simulink library "EVComponents_utility_lib"  (R2021a)
settings: Solver=VariableStepAuto  StartTime=0.0  StopTime=10.0  RelTol=1e-3
undefined symbols (not defined in the file): DiscIntNeverNeededParam
libraries: fl_lib x7, nesl_utility x5, $bdroot x1, sdl_lib x1
settings Model: Creator=isaacito  LastModifiedBy=isaacito
settings SolverCC: AlgebraicLoopSolver=TrustRegion
settings DebuggingCC: SFMachineParentedDataDiag=warning

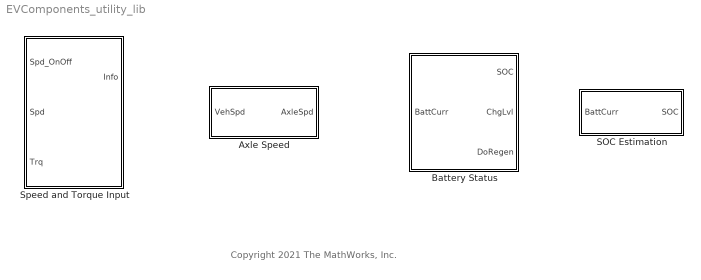
== system EVComponents_utility_lib ==
  note: Copyright 2021 The MathWorks, Inc.
  Axle Speed : Subsystem  mask(Vehicle Speed to Axle Speed){Value=0.3}
      mask prompts: Value "Tire Rolling Radius [m]"
      mask help: Given longitudinal vehicle speed, this block computes the axle rotational speed.
      mask TypeOptions Value: Tire Rolling Radius (m)/Value
  Battery Status : Subsystem  mask(Battery Status){capacity_kWh=40, voltagePerCell_V=3.5, initial_SOC_pct=98, SocHigh=95, SocLow=50, SocEmpty=6}
      mask prompts: capacity_kWh "Battery Capacity [kW*hr]"; voltagePerCell_V "Voltage per cell [V]"; initial_SOC_pct "Initial SOC [%]"; SocHigh "SOC High-Mid Threshold [%]"; SocLow "SOC Mid-Low Threshold [%]"; SocEmpty "SOC Low-Empty Threshold [%]"
      mask help:
      | Battery current input assumes that the negative (positive) value current means consuming (charging) electric power from (to) the battery.
      |
      | SOC outport outputs the state of charge of the battery in %.
      |
      | ChgLvl outport outputs the charge levels 0 (empty), 1 (low), 2 (mid), or 3 (high). Specify thresholds in SOC Threshold parameters.
      |
      | DoRegen outport outputs true for empty/low/mid battery charge level and false for high. Use this signal to avoid overcharging the battery.
      mask init:
      | if initial_SOC_pct > SocHigh
      |   initialChgLvl = 3;
      | elseif initial_SOC_pct < SocEmpty
      |   initialChgLvl = 0;
      | elseif initial_SOC_pct > SocLow
      |   initialChgLvl = 2;
      | else
      |   initialChgLvl = 1;
      | end
      mask TypeOptions capacity_kWh: SOC Estimation/capacity_kWh
      mask TypeOptions voltagePerCell_V: SOC Estimation/voltagePerCell_V
      mask TypeOptions initial_SOC_pct: SOC Estimation/initial_SOC_pct
      mask DialogControl Container2 Prompt: Parameters
  SOC Estimation : Subsystem  mask(Battery State-of-Charge Estimation){capacity_kWh=10, voltagePerCell_V=3.5, initial_SOC_pct=90}
      mask prompts: capacity_kWh "Battery Capacity [kW*hr]"; voltagePerCell_V "Voltage per cell [V]"; initial_SOC_pct "Initial SOC [%]"
      mask help: Battery current input assumes that the negative value current meas consuming electric power from the battery.
      mask TypeOptions capacity_kWh: Capacity (kW*hr)/Value
      mask TypeOptions voltagePerCell_V: Voltage per Cell (V)/Value
      mask TypeOptions initial_SOC_pct: Initial SOC (%)/Value
  Speed and Torque Input : Subsystem  mask(Speed and Torque Input){t_friction=10000, t_locked=10000, w_tol=0.001, initial_state_locked=sdl.enum.initial_lock.unlocked}
      mask prompts: t_friction "Kinetic friction torque [N*m]"; t_locked "Static friction torque [N*m]"; w_tol "Clutch velocity tolerance [rad/s]"; initial_state_locked "Initial state"
      mask help:
      | This block acts as angular speed and torque source for Simscape Mechanical Rotational connection. Pass 0 or 1 at Spd_OnOff inport to disable or enable speed input Spd, respectively.
      |
      | Spd inport takes angular speed in rpm. Trq inport takes torques in N*m. Node R is Simscape Mechanical Rotational connection node. Info outport outputs angular speed and torque at R.
      |
      | Block parameters correspond to the Logic-Controlled Clutch block in Simscape Driveline.
      mask TypeOptions t_friction:
      | Logic-Controlled
      | Clutch/t_friction
      mask TypeOptions t_locked:
      | Logic-Controlled
      | Clutch/t_locked
      mask TypeOptions w_tol:
      | Logic-Controlled
      | Clutch/w_tol
      mask TypeOptions initial_state_locked:
      | Logic-Controlled
      | Clutch/initial_state_locked

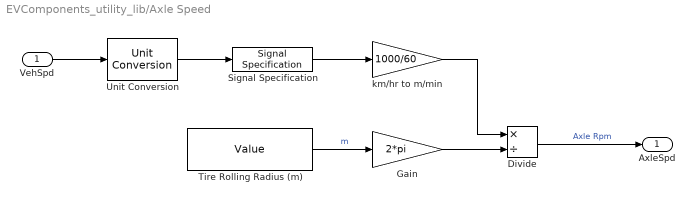
== system EVComponents_utility_lib/Axle Speed ==
  VehSpd : Inport
      settings: AttributesFormatString=%<Unit>
  Divide : Product  Inputs=*/
  Gain : Gain  Gain=2*pi
  Signal Specification : SignalSpecification  Unit=km/hr
  Tire Rolling Radius (m) : Constant  Value=Value
  Unit Conversion : UnitConversion
  km/hr to m/min : Gain  Gain=1000/60
  AxleSpd : Outport  Unit=rpm  VectorParamsAs1DForOutWhenUnconnected=off
      settings: AttributesFormatString=%<Unit>
  wires:
  Tire Rolling Radius (m)/1 -> Gain/1  "m"
  Gain/1 -> Divide/2
  Divide/1 -> AxleSpd/1  "Axle Rpm"
  Unit Conversion/1 -> Signal Specification/1
  VehSpd/1 -> Unit Conversion/1
  Signal Specification/1 -> km/hr to m/min/1
  km/hr to m/min/1 -> Divide/1

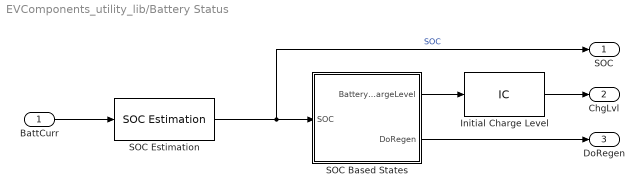
== system EVComponents_utility_lib/Battery Status ==
  BattCurr : Inport
  Initial Charge Level : InitialCondition  Value=initialChgLvl
  SOC Based States : Stateflow chart  TreatAsAtomicUnit=on
      settings: PortSchema="{\"entries\":[{\"content\":{\"sides\":[{\"content\":{\"connectorIds\":[\"In1\"]},\"type\":\"ConnectorPlacement.EquallySpacedRectSide\",\"uuid\":\"6842a8e0-1533-443f-9239-a32cee073609\"},{\"content\":{\"connectorIds\":[\"Out2\",\"Out1\"],\"side\":\"RIGHT\"},\"type\":\"ConnectorPlacement.EquallySpacedRectSide\",\"uuid\":\"4d5668fa-96aa-414a-86e2-97093b53d80f\"},{\"content\":{\"connectorIds\":[],\"side\":\"TOP\"},\"type\":\"ConnectorPlacement.EquallySpacedRectSide\",\"uuid\":\"b14b12e5-8ddb-4090-8868-1deded7232d1\"},{\"content\":{\"connectorIds\":[],\"side\":\"HIDDEN\"},\"type\":\"ConnectorPlacement.EquallySpacedRectSide\",\"uuid\":\"15641086-7bcd-4523-b266-ad823dacae84\"}]},\"type\":\"ConnectorPlacement.EquallySpacedConnector\",\"uuid\":\"9c75feda-b5f3-44ec-8ad2-652491ceb2eb\"}],\"packageUris\":[\"http://schema.mathworks.com/mf0/Connector/R2020b\"],\"version\":\"1.0\"}"
  SOC Estimation : $bdroot/SOC Estimation  capacity_kWh=capacity_kWh  voltagePerCell_V=voltagePerCell_V  initial_SOC_pct=initial_SOC_pct
  SOC : Outport
  ChgLvl : Outport  Port=2
  DoRegen : Outport  Port=3
  wires:
  SOC Estimation/1 -> SOC/1, SOC Based States/1(SOC)  "SOC"
  SOC Based States/1(DoRegen) -> DoRegen/1
  SOC Based States/2(BatteryChargeLevel) -> Initial Charge Level/1
  BattCurr/1 -> SOC Estimation/1
  Initial Charge Level/1 -> ChgLvl/1

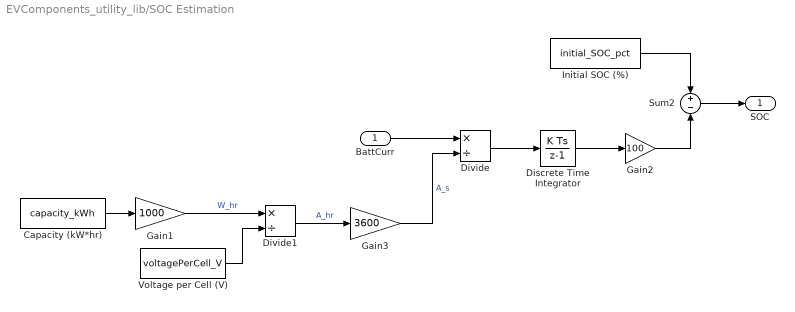
== system EVComponents_utility_lib/SOC Estimation ==
  BattCurr : Inport  Unit=A
      settings: AttributesFormatString=%<Unit>
  Capacity (kW*hr) : Constant  Value=capacity_kWh
  Discrete Time Integrator : DiscreteIntegrator  SampleTime=-1  ICPrevOutput=DiscIntNeverNeededParam  ICPrevScaledInput=DiscIntNeverNeededParam
  Divide : Product  Inputs=*/
  Divide1 : Product  Inputs=*/
  Gain1 : Gain  Gain=1000
  Gain2 : Gain  Gain=100
  Gain3 : Gain  Gain=3600
  Initial SOC (%) : Constant  Value=initial_SOC_pct
  Sum2 : Sum  Inputs=+-
  Voltage per Cell (V) : Constant  Value=voltagePerCell_V
  SOC : Outport  Unit=%
      settings: AttributesFormatString=%<Unit>
  wires:
  Sum2/1 -> SOC/1
  Initial SOC (%)/1 -> Sum2/1
  Discrete Time Integrator/1 -> Gain2/1
  Divide/1 -> Discrete Time Integrator/1
  Gain2/1 -> Sum2/2
  Gain3/1 -> Divide/2  "A_s"
  BattCurr/1 -> Divide/1
  Divide1/1 -> Gain3/1  "A_hr"
  Voltage per Cell (V)/1 -> Divide1/2
  Capacity (kW*hr)/1 -> Gain1/1
  Gain1/1 -> Divide1/1  "W_hr"

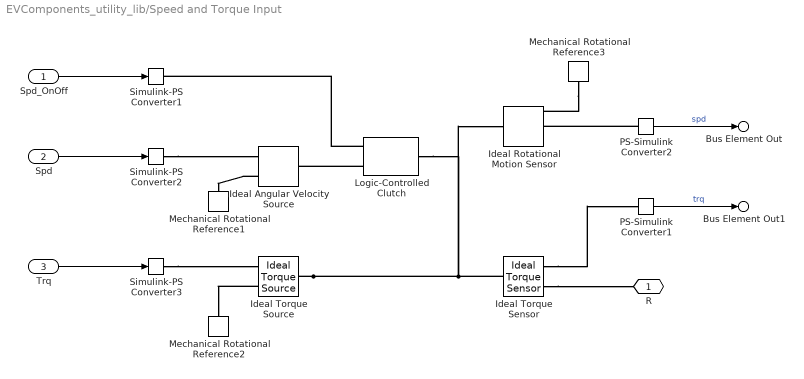
== system EVComponents_utility_lib/Speed and Torque Input ==
  Spd_OnOff : Inport  Unit=1
      settings: AttributesFormatString=%<Unit>
  Spd : Inport  Port=2  Unit=rpm
      settings: AttributesFormatString=%<Unit>
  Trq : Inport  Port=3  Unit=N*m
      settings: AttributesFormatString=%<Unit>
  Ideal Angular Velocity Source : fl_lib/Mechanical/Mechanical Sources/Ideal Angular Velocity Source
  Ideal Rotational Motion Sensor : fl_lib/Mechanical/Mechanical Sensors/Ideal Rotational Motion Sensor  wrap_angle=simscape.enum.onoff.off  offset=0 rad
  Ideal Torque Sensor : fl_lib/Mechanical/Mechanical Sensors/Ideal Torque Sensor
  Ideal Torque Source : fl_lib/Mechanical/Mechanical Sources/Ideal Torque Source
  Logic-Controlled Clutch : sdl_lib/Clutches/Logic-Controlled Clutch  t_friction=t_friction N*m  t_locked=t_locked N*m  w_tol=w_tol rad/s  initial_state_locked=initial_state_locked
      settings: SourceProductBaseCode=LD  InternalSimscapePortConfiguration="{\"Bottom\":[],\"Left\":[{\"id\":\"E\",\"label\":\"E\",\"type\":\"input\"},{\"id\":\"B\",\"label\":\"B\",\"type\":\"foundation.mechanical.rotational.rotational\"}],\"Right\":[{\"id\":\"F\",\"label\":\"F\",\"type\":\"foundation.mechanical.rotational.rotational\"}],\"Top\":[]}"
  Mechanical Rotational Reference1 : fl_lib/Mechanical/Rotational Elements/Mechanical Rotational Reference
  Mechanical Rotational Reference2 : fl_lib/Mechanical/Rotational Elements/Mechanical Rotational Reference
  Mechanical Rotational Reference3 : fl_lib/Mechanical/Rotational Elements/Mechanical Rotational Reference
  PS-Simulink Converter1 : nesl_utility/PS-Simulink Converter  PhysicalDomain=network_engine_domain  SubClassName=ps_output  LeftPortType=input  RightPortType=output  PseudoPeriodic=off  Frequencies=[]  Unit=N*m  AffineConversion=off
      settings: SourceProductBaseCode=PW,SS
  PS-Simulink Converter2 : nesl_utility/PS-Simulink Converter  PhysicalDomain=network_engine_domain  SubClassName=ps_output  LeftPortType=input  RightPortType=output  PseudoPeriodic=off  Frequencies=[]  Unit=rpm  AffineConversion=off
      settings: SourceProductBaseCode=PW,SS
  Simulink-PS Converter1 : nesl_utility/Simulink-PS Converter  PhysicalDomain=network_engine_domain  SubClassName=ps_input  LeftPortType=input  RightPortType=output  PseudoPeriodic=off  Frequencies=[]  NoiseDistribution=none  NoiseParameters=[]  Unit=1  AffineConversion=off  FilteringAndDerivatives=provide  SimscapeFilterOrder=1  InputFilterTimeConstant=0.001  UdotUserProvided=0
      settings: SourceProductBaseCode=PW,SS
  Simulink-PS Converter2 : nesl_utility/Simulink-PS Converter  PhysicalDomain=network_engine_domain  SubClassName=ps_input  LeftPortType=input  RightPortType=output  PseudoPeriodic=off  Frequencies=[]  NoiseDistribution=none  NoiseParameters=[]  Unit=rpm  AffineConversion=off  FilteringAndDerivatives=filter  SimscapeFilterOrder=1  InputFilterTimeConstant=0.001  UdotUserProvided=0
      settings: SourceProductBaseCode=PW,SS
  Simulink-PS Converter3 : nesl_utility/Simulink-PS Converter  PhysicalDomain=network_engine_domain  SubClassName=ps_input  LeftPortType=input  RightPortType=output  PseudoPeriodic=off  Frequencies=[]  NoiseDistribution=none  NoiseParameters=[]  Unit=N*m  AffineConversion=off  FilteringAndDerivatives=filter  SimscapeFilterOrder=1  InputFilterTimeConstant=0.001  UdotUserProvided=0
      settings: SourceProductBaseCode=PW,SS
  R : PMIOPort  Side=Right
  Bus Element Out : Outport  PortName=Info  Element=spd
  Bus Element Out1 : Outport  PortName=Info  Element=trq
  wires:
  Spd/1 -> Simulink-PS Converter2/1
  Spd_OnOff/1 -> Simulink-PS Converter1/1
  Trq/1 -> Simulink-PS Converter3/1
  PS-Simulink Converter1/1 -> Bus Element Out1/1  "trq"
  PS-Simulink Converter2/1 -> Bus Element Out/1  "spd"
  connections:
  Logic-Controlled Clutch/LConn1 -- Simulink-PS Converter1/RConn1
  Ideal Torque Source/RConn2 -- Mechanical Rotational Reference2/LConn1
  Ideal Torque Sensor/RConn1 -- R/RConn1
  Logic-Controlled Clutch/LConn2 -- Ideal Angular Velocity Source/LConn1
  Ideal Angular Velocity Source/RConn2 -- Mechanical Rotational Reference1/LConn1
  Simulink-PS Converter2/RConn1 -- Ideal Angular Velocity Source/RConn1
  Simulink-PS Converter3/RConn1 -- Ideal Torque Source/RConn1
  Ideal Torque Source/LConn1 -- Ideal Torque Sensor/LConn1 -- Logic-Controlled Clutch/RConn1 -- Ideal Rotational Motion Sensor/LConn1
  PS-Simulink Converter2/LConn1 -- Ideal Rotational Motion Sensor/RConn2
  Mechanical Rotational Reference3/LConn1 -- Ideal Rotational Motion Sensor/RConn1
  Ideal Torque Sensor/RConn2 -- PS-Simulink Converter1/LConn1

== stateflow chart EVComponents_utility_lib/Battery Status/SOC Based States ==
  state SocHigh
    entry:
    BatteryChargeLevel = 3;
    DoRegen = false;
  state Classify
  state SocOk
    entry:
    BatteryChargeLevel = 2;
    DoRegen = true;
  state SocLow
    entry:
    BatteryChargeLevel = 1;
    DoRegen = true;
  state SocEmpty
    entry:
    BatteryChargeLevel = 0;
    DoRegen = true;
  (junction 11) -> SocHigh : [ SocHigh <= SOC ]
  Classify -> (junction 11) [order 1]
  SocOk -> SocHigh [order 1] : [ SocHigh + 2 < SOC ]
  SocHigh -> SocOk : [ SOC < SocHigh - 2 ]
  Classify -> SocOk [order 2] : [ SocLow <= SOC & SOC < SocHigh ]
  (default) -> Classify
  Classify -> (junction 31) [order 4]
  Classify -> (junction 15) [order 3]
  SocLow -> SocOk [order 1] : [ SocLow + 2 < SOC ]
  SocOk -> SocLow [order 2] : [ SOC < SocLow - 2 ]
  (junction 15) -> SocLow : [ SocEmpty <= SOC & SOC < SocLow ]
  SocEmpty -> SocLow : [ SocEmpty + 1 < SOC ]
  SocLow -> SocEmpty [order 2] : [ SOC < SocEmpty - 1 ]
  (junction 31) -> SocEmpty : [ SOC < SocEmpty ]
  data: SOC input; SocLow parameter double; SocHigh parameter double; DoRegen output; BatteryChargeLevel output; SocEmpty parameter
